simulink model "Loop_spring_mass_damper_system"  (R2022b)
settings: Solver=FixedStepAuto  StartTime=0  StopTime=Tf  FixedStep=dt  RelTol=1e-3
values from neighbouring files (symbols this model uses):
  c = 1    [Loop_slx_main.m]
  control_on = true    [Loop_slx_main.m]
  control_period = 0.1    [Loop_slx_main.m]
  disturbance_on = false    [Loop_slx_main.m]
  k = 10    [Loop_slx_main.m]
  Kp = 10    [Loop_slx_main.m]
  m = 1    [Loop_slx_main.m]
  omega_1 = 0.1    [Loop_slx_main.m]
  omega_3 = 8    [Loop_slx_main.m]
  omega_4 = 0.5    [Loop_slx_main.m]
  r = [0 0]'    [Loop_slx_main.m]
  v0 = 0    [Loop_slx_main.m]
  x0 = 1    [Loop_slx_main.m]
libraries: dspsrcs4 x1
settings Model: Creator=murayama  LastModifiedBy=murayama
settings DataIOCC: SaveFormat=StructureWithTime  ReturnWorkspaceOutputs=off
settings OptimizationCC: BlockReduction=off  BufferReuse=off
settings DebuggingCC: AlgebraicLoopMsg=none

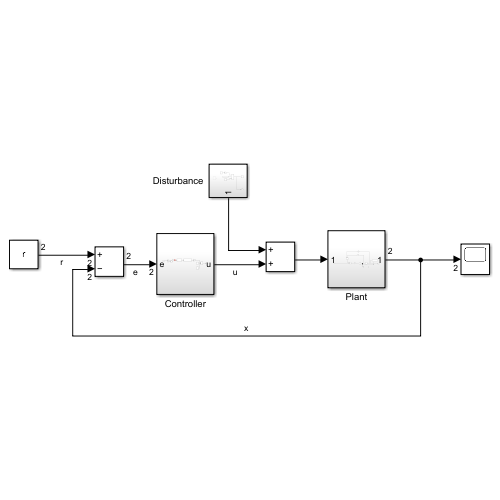
[thumbnail: Simulink's stored preview of the top-level diagram]
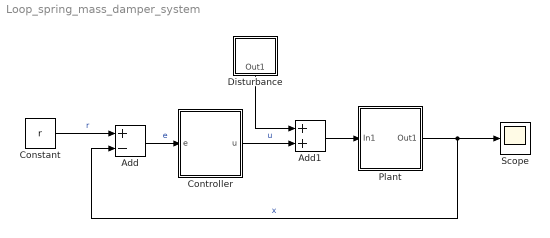
== system Loop_spring_mass_damper_system ==
  Add : Sum  Inputs=+-
  Add1 : Sum
  Constant : Constant  Value=r
  Controller : Subsystem
  Disturbance : Subsystem
  Plant : Subsystem
  Scope : Scope
  wires:
  Plant/1(Out1) -> Add/2, Scope/1  "x"
  Constant/1 -> Add/1  "r"
  Add/1 -> Controller/1(e)  "e"
  Add1/1 -> Plant/1(In1)
  Disturbance/1(Out1) -> Add1/1
  Controller/1(u) -> Add1/2  "u"

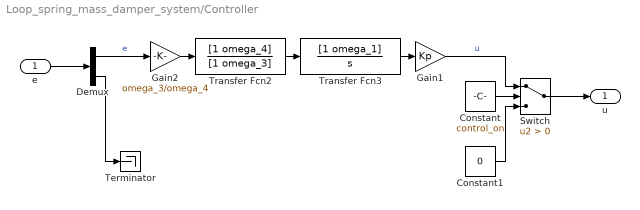
== system Loop_spring_mass_damper_system/Controller ==
  e : Inport
  Constant : Constant  Value=control_on
  Constant1 : Constant  Value=0
  Demux : Demux  Outputs=2
  Gain1 : Gain  Gain=Kp
  Gain2 : Gain  Gain=omega_3/omega_4
  Switch : Switch  Criteria=u2 > Threshold  SaturateOnIntegerOverflow=off  InputSameDT=off
  Terminator : Terminator
  Transfer Fcn2 : TransferFcn  Numerator=[1 omega_4]  Denominator=[1 omega_3]
  Transfer Fcn3 : TransferFcn  Numerator=[1 omega_1]  Denominator=[1 0]
  u : Outport
  wires:
  Gain1/1 -> Switch/1  "u"
  e/1 -> Demux/1
  Constant/1 -> Switch/2
  Switch/1 -> u/1
  Constant1/1 -> Switch/3
  Transfer Fcn2/1 -> Transfer Fcn3/1
  Gain2/1 -> Transfer Fcn2/1
  Transfer Fcn3/1 -> Gain1/1
  Demux/1 -> Gain2/1  "e"
  Demux/2 -> Terminator/1

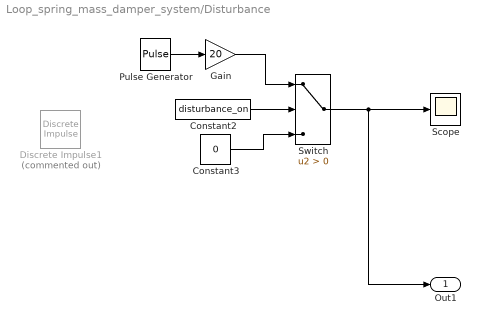
== system Loop_spring_mass_damper_system/Disturbance ==
  Constant2 : Constant  Value=disturbance_on
  Constant3 : Constant  Value=0
  Discrete Impulse1 : dspsrcs4/Discrete  Impulse  Commented=on  Delay=0  SampleTime=control_period  FrameSample=1  OutputFrames=off  dataType=double  isSigned=on  wordLen=16  udDataType=sfix(16)  fracBitsMode=Best precision  numFracBits=15  OutDataTypeStr=double  LastOutDataTypeStr=double
  Gain : Gain  Gain=20
  Pulse Generator : DiscretePulseGenerator  Period=100  PulseWidth=10  PhaseDelay=20  SampleTime=control_period
  Scope : Scope
  Switch : Switch  Criteria=u2 > Threshold  SaturateOnIntegerOverflow=off  InputSameDT=off
  Out1 : Outport
  wires:
  Constant3/1 -> Switch/3
  Switch/1 -> Scope/1, Out1/1
  Gain/1 -> Switch/1
  Pulse Generator/1 -> Gain/1
  Constant2/1 -> Switch/2

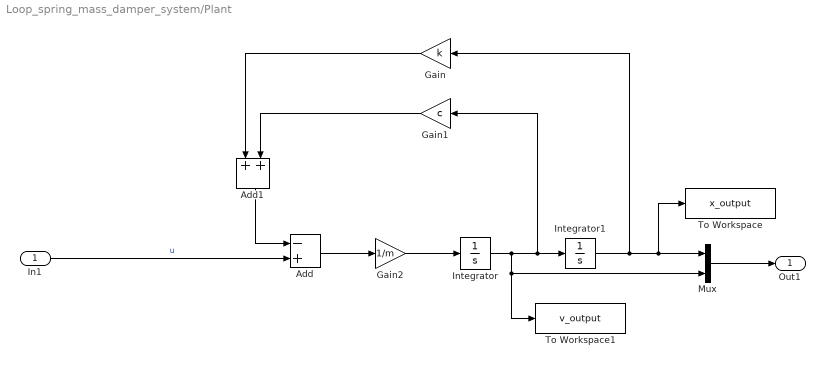
== system Loop_spring_mass_damper_system/Plant ==
  In1 : Inport
  Add : Sum  Inputs=-+
  Add1 : Sum
  Gain : Gain  Gain=k
  Gain1 : Gain  Gain=c
  Gain2 : Gain  Gain=1/m
  Integrator : Integrator  InitialCondition=v0
  Integrator1 : Integrator  InitialCondition=x0
  Mux : Mux  Inputs=2
  To Workspace : ToWorkspace  VariableName=x_output  SaveFormat=Timeseries  SampleTime=-1
  To Workspace1 : ToWorkspace  VariableName=v_output  SaveFormat=Timeseries  SampleTime=-1
  Out1 : Outport
  wires:
  Integrator1/1 -> Gain/1, To Workspace/1, Mux/1
  Add1/1 -> Add/1
  Gain/1 -> Add1/1
  Add/1 -> Gain2/1
  Gain2/1 -> Integrator/1
  Integrator/1 -> To Workspace1/1, Mux/2, Gain1/1, Integrator1/1
  Gain1/1 -> Add1/2
  In1/1 -> Add/2  "u"
  Mux/1 -> Out1/1
